simulink model "msiglabel_out"  (Simulink 6.3)
settings: Solver=FixedStepDiscrete  StartTime=0.0  StopTime=10.0  RelTol=1e-3
settings Model: Creator=awarlock  LastModifiedBy=mshakeri  ExtModeAutoUpdateStatusClock=off  StrictBusMsg=ErrorLevel1
settings OptimizationCC: InlineParams=on  InlineInvariantSignals=on
settings DebuggingCC: CheckExecutionContextPreStartOutputMsg=on  CheckExecutionContextRuntimeOutputMsg=on  SolverPrmCheckMsg=none  UnconnectedInputMsg=none  UnconnectedOutputMsg=none  UnconnectedLineMsg=none

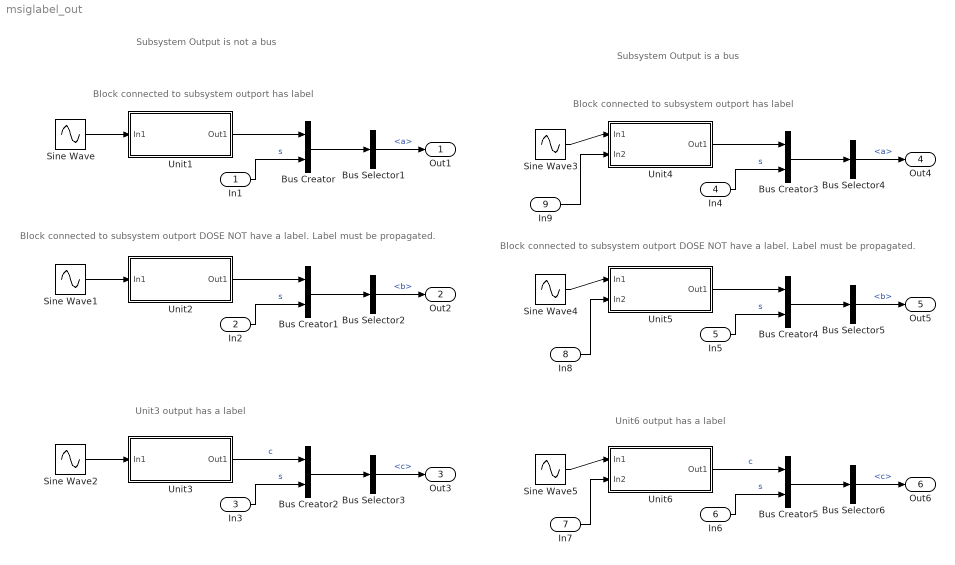
== system msiglabel_out ==
  note: Block connected to subsystem outport has label
  note: Block connected to subsystem outport DOSE NOT have a label.
      | Label must be propagated.
  note: Unit3 output has a label
  note: Block connected to subsystem outport has label
  note: Block connected to subsystem outport DOSE NOT have a label.
      | Label must be propagated.
  note: Unit6 output has a label
  note: Subsystem Output is not a bus
  note: Subsystem Output is a bus
  In1 : Inport  Port=1  LatchInput=off
  In2 : Inport  Port=2  LatchInput=off
  In3 : Inport  Port=3  LatchInput=off
  In4 : Inport  Port=4  LatchInput=off
  In5 : Inport  Port=5  LatchInput=off
  In6 : Inport  Port=6  LatchInput=off
  In7 : Inport  Port=7  LatchInput=off
  In8 : Inport  Port=8  LatchInput=off
  In9 : Inport  Port=9  LatchInput=off
  Bus Creator{,1..5} (6 alike) : BusCreator  Inputs=2
  Bus Selector1 : BusSelector  OutputSignals=a
  Bus Selector2 : BusSelector  OutputSignals=b
  Bus Selector3 : BusSelector  OutputSignals=c
  Bus Selector4 : BusSelector  OutputSignals=a
  Bus Selector5 : BusSelector  OutputSignals=b
  Bus Selector6 : BusSelector  OutputSignals=c
  Sine Wave{,1..5} (6 alike) : Sin  SampleTime=0
  Unit1 : Subsystem  TreatAsAtomicUnit=on
  Unit2 : Subsystem  TreatAsAtomicUnit=on
  Unit3 : Subsystem  TreatAsAtomicUnit=on
  Unit4 : Subsystem  TreatAsAtomicUnit=on
  Unit5 : Subsystem  TreatAsAtomicUnit=on
  Unit6 : Subsystem  TreatAsAtomicUnit=on
  Out1 : Outport
  Out2 : Outport  Port=2
  Out3 : Outport  Port=3
  Out4 : Outport  Port=4
  Out5 : Outport  Port=5
  Out6 : Outport  Port=6
  wires:
  Bus Creator/1 -> Bus Selector1/1
  Sine Wave/1 -> Unit1/1(In1)
  Unit1/1(Out1) -> Bus Creator/1
  In1/1 -> Bus Creator/2  "s"
  Bus Creator1/1 -> Bus Selector2/1
  Sine Wave1/1 -> Unit2/1(In1)
  Unit2/1(Out1) -> Bus Creator1/1
  In2/1 -> Bus Creator1/2  "s"
  Bus Selector1/1 -> Out1/1  "<a>"
  Bus Selector2/1 -> Out2/1  "<b>"
  Bus Creator2/1 -> Bus Selector3/1
  Sine Wave2/1 -> Unit3/1(In1)
  Unit3/1(Out1) -> Bus Creator2/1  "c"
  In3/1 -> Bus Creator2/2  "s"
  Bus Selector3/1 -> Out3/1  "<c>"
  Bus Creator3/1 -> Bus Selector4/1
  Sine Wave3/1 -> Unit4/1(In1)
  Unit4/1(Out1) -> Bus Creator3/1
  In4/1 -> Bus Creator3/2  "s"
  Bus Creator4/1 -> Bus Selector5/1
  Sine Wave4/1 -> Unit5/1(In1)
  Unit5/1(Out1) -> Bus Creator4/1
  In5/1 -> Bus Creator4/2  "s"
  Bus Selector4/1 -> Out4/1  "<a>"
  Bus Selector5/1 -> Out5/1  "<b>"
  Bus Creator5/1 -> Bus Selector6/1
  Sine Wave5/1 -> Unit6/1(In1)
  Unit6/1(Out1) -> Bus Creator5/1  "c"
  In6/1 -> Bus Creator5/2  "s"
  Bus Selector6/1 -> Out6/1  "<c>"
  In7/1 -> Unit6/2(In2)
  In8/1 -> Unit5/2(In2)
  In9/1 -> Unit4/2(In2)

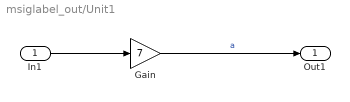
== system msiglabel_out/Unit1 ==
  In1 : Inport  Port=1  LatchInput=off
  Gain : Gain  Gain=7
  Out1 : Outport
  wires:
  In1/1 -> Gain/1
  Gain/1 -> Out1/1  "a"

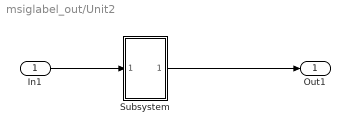
== system msiglabel_out/Unit2 ==
  In1 : Inport  Port=1  LatchInput=off
  Subsystem : Subsystem
  Out1 : Outport
  wires:
  Subsystem/1(Out1) -> Out1/1
  In1/1 -> Subsystem/1(In1)

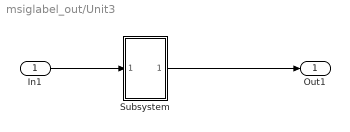
== system msiglabel_out/Unit3 ==
  In1 : Inport  Port=1  LatchInput=off
  Subsystem : Subsystem
  Out1 : Outport
  wires:
  In1/1 -> Subsystem/1(In1)
  Subsystem/1(Out1) -> Out1/1

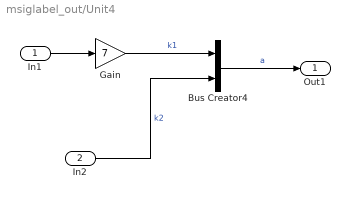
== system msiglabel_out/Unit4 ==
  In1 : Inport  Port=1  LatchInput=off
  In2 : Inport  Port=2  LatchInput=off
  Bus Creator4 : BusCreator  Inputs=2
  Gain : Gain  Gain=7
  Out1 : Outport
  wires:
  In1/1 -> Gain/1
  Bus Creator4/1 -> Out1/1  "a"
  Gain/1 -> Bus Creator4/1  "k1"
  In2/1 -> Bus Creator4/2  "k2"

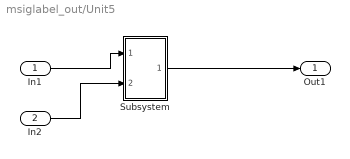
== system msiglabel_out/Unit5 ==
  In1 : Inport  Port=1  LatchInput=off
  In2 : Inport  Port=2  LatchInput=off
  Subsystem : Subsystem
  Out1 : Outport
  wires:
  Subsystem/1(Out1) -> Out1/1
  In1/1 -> Subsystem/1(In1)
  In2/1 -> Subsystem/2(In2)

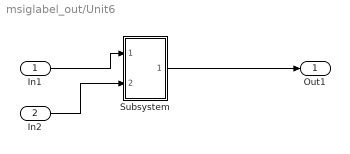
== system msiglabel_out/Unit6 ==
  In1 : Inport  Port=1  LatchInput=off
  In2 : Inport  Port=2  LatchInput=off
  Subsystem : Subsystem
  Out1 : Outport
  wires:
  In1/1 -> Subsystem/1(In1)
  Subsystem/1(Out1) -> Out1/1
  In2/1 -> Subsystem/2(In2)

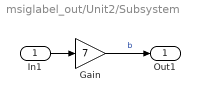
== system msiglabel_out/Unit2/Subsystem ==
  In1 : Inport  Port=1  LatchInput=off
  Gain : Gain  Gain=7
  Out1 : Outport
  wires:
  In1/1 -> Gain/1
  Gain/1 -> Out1/1  "b"

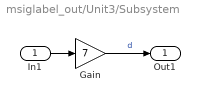
== system msiglabel_out/Unit3/Subsystem ==
  In1 : Inport  Port=1  LatchInput=off
  Gain : Gain  Gain=7
  Out1 : Outport
  wires:
  Gain/1 -> Out1/1  "d"
  In1/1 -> Gain/1

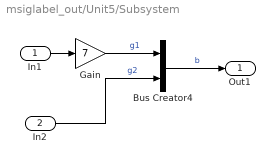
== system msiglabel_out/Unit5/Subsystem ==
  In1 : Inport  Port=1  LatchInput=off
  In2 : Inport  Port=2  LatchInput=off
  Bus Creator4 : BusCreator  Inputs=2
  Gain : Gain  Gain=7
  Out1 : Outport
  wires:
  In1/1 -> Gain/1
  Gain/1 -> Bus Creator4/1  "g1"
  Bus Creator4/1 -> Out1/1  "b"
  In2/1 -> Bus Creator4/2  "g2"

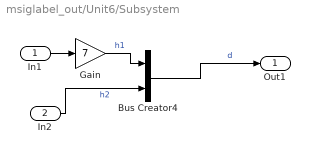
== system msiglabel_out/Unit6/Subsystem ==
  In1 : Inport  Port=1  LatchInput=off
  In2 : Inport  Port=2  LatchInput=off
  Bus Creator4 : BusCreator  Inputs=2
  Gain : Gain  Gain=7
  Out1 : Outport
  wires:
  In1/1 -> Gain/1
  Gain/1 -> Bus Creator4/1  "h1"
  In2/1 -> Bus Creator4/2  "h2"
  Bus Creator4/1 -> Out1/1  "d"
